simulink model "SolarTrackerModelRoboticsAss"  (R2024b)
settings: Solver=VariableStepAuto  StartTime=0.0  StopTime=10.0  RelTol=1e-3
libraries: simulink x1
settings Model: Creator=MY LAPTOP  LastModifiedBy=MY LAPTOP

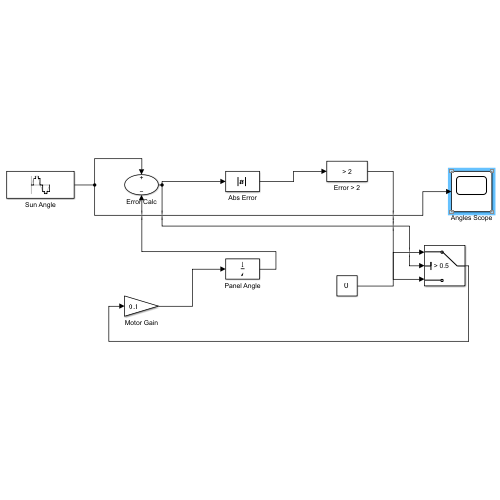
[thumbnail: Simulink's stored preview of the top-level diagram]
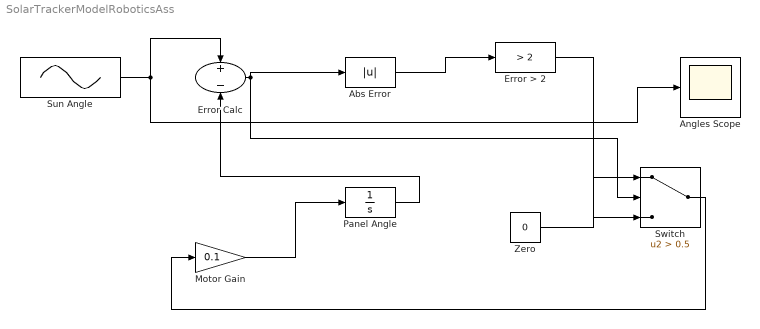
== system SolarTrackerModelRoboticsAss ==
  Abs Error : Abs  SaturateOnIntegerOverflow=off
  Angles Scope : Scope
  Error > 2 : simulink/Logic and Bit Operations/Compare To Constant  relop=>  const=2  OutDataTypeStr=boolean
  Error Calc : Sum  Inputs=+-
  Motor Gain : Gain  Gain=0.1
  Panel Angle : Integrator
  Sun Angle : Sin  Amplitude=90  Bias=90  Frequency=2*pi/86400  SampleTime=1
  Switch : Switch  Criteria=u2 > Threshold  Threshold=0.5  SaturateOnIntegerOverflow=off  InputSameDT=off
  Zero : Constant  Value=0
  wires:
  Sun Angle/1 -> Angles Scope/1, Error Calc/1
  Panel Angle/1 -> Error Calc/2
  Error Calc/1 -> Switch/2, Abs Error/1
  Abs Error/1 -> Error > 2/1
  Error > 2/1 -> Switch/3
  Zero/1 -> Switch/1
  Switch/1 -> Motor Gain/1
  Motor Gain/1 -> Panel Angle/1
